simulink model "controlador"  (R2021a)
settings: Solver=ode4  StartTime=0.0  StopTime=2  FixedStep=10e-3  RelTol=1e-3
values from neighbouring files (symbols this model uses):
  ka = k/kt    (= 86.7924528302)    [parametros_controlador.m]
  ki_crit = 1/(4*k*tau)    (= 2.15153705807)    [parametros_controlador.m]
  ki_sub = (wn^2*tau)/(ka*kt)    [parametros_controlador.m]
  kp = 1/k    (= 0.724637681159)    [parametros_controlador.m]
  kt = 0.0159    [parametros_controlador.m]
  tau = 0.0842    [parametros_controlador.m]
  Ti = 1/z    (= 0.0592540464462)    [parametros_controlador.m]
settings Model: Creator=Isabella  LastModifiedBy=Usuário

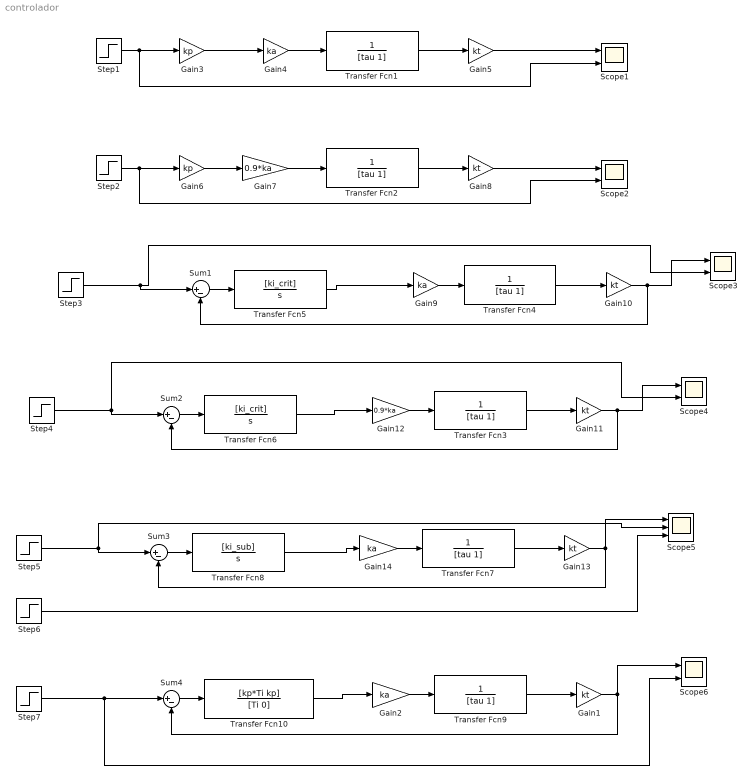
== system controlador ==
  Gain{1,5,8,10..11,13} (6 alike) : Gain  Gain=kt
  Gain12 : Gain  Gain=0.9*ka
  Gain{2,4,9,14} (4 alike) : Gain  Gain=ka
  Gain3 : Gain  Gain=kp
  Gain6 : Gain  Gain=kp
  Gain7 : Gain  Gain=0.9*ka
  Scope{1..4,6} (5 alike) : Scope  NumInputPorts=2
  Scope5 : Scope  NumInputPorts=3
  Step{1..5,7} (6 alike) : Step  Time=0  After=10  SampleTime=0
  Step6 : Step  Time=0  After=10*1.05  SampleTime=0
  Sum{1..4} (4 alike) : Sum  Inputs=|+-
  Transfer Fcn{1..4,7,9} (6 alike) : TransferFcn  Denominator=[tau 1]
  Transfer Fcn10 : TransferFcn  Numerator=[kp*Ti kp]  Denominator=[Ti 0]
  Transfer Fcn5 : TransferFcn  Numerator=[ki_crit]  Denominator=[1 0]
  Transfer Fcn6 : TransferFcn  Numerator=[ki_crit]  Denominator=[1 0]
  Transfer Fcn8 : TransferFcn  Numerator=[ki_sub]  Denominator=[1 0]
  wires:
  Step1/1 -> Scope1/2, Gain3/1
  Gain5/1 -> Scope1/1
  Gain4/1 -> Transfer Fcn1/1
  Gain3/1 -> Gain4/1
  Transfer Fcn1/1 -> Gain5/1
  Transfer Fcn2/1 -> Gain8/1
  Gain6/1 -> Gain7/1
  Gain8/1 -> Scope2/1
  Step2/1 -> Scope2/2, Gain6/1
  Gain7/1 -> Transfer Fcn2/1
  Gain10/1 -> Sum1/2, Scope3/1
  Step3/1 -> Sum1/1, Scope3/2
  Gain9/1 -> Transfer Fcn4/1
  Sum1/1 -> Transfer Fcn5/1
  Transfer Fcn4/1 -> Gain10/1
  Transfer Fcn5/1 -> Gain9/1
  Transfer Fcn6/1 -> Gain12/1
  Transfer Fcn3/1 -> Gain11/1
  Gain12/1 -> Transfer Fcn3/1
  Step4/1 -> Sum2/1, Scope4/2
  Sum2/1 -> Transfer Fcn6/1
  Gain11/1 -> Sum2/2, Scope4/1
  Transfer Fcn8/1 -> Gain14/1
  Transfer Fcn7/1 -> Gain13/1
  Gain13/1 -> Sum3/2, Scope5/1
  Sum3/1 -> Transfer Fcn8/1
  Step5/1 -> Sum3/1, Scope5/2
  Gain14/1 -> Transfer Fcn7/1
  Step6/1 -> Scope5/3
  Gain2/1 -> Transfer Fcn9/1
  Step7/1 -> Scope6/2, Sum4/1
  Transfer Fcn10/1 -> Gain2/1
  Sum4/1 -> Transfer Fcn10/1
  Gain1/1 -> Sum4/2, Scope6/1
  Transfer Fcn9/1 -> Gain1/1
